simulink model "parte5_eje1_Ks"  (R2019b)
settings: Solver=VariableStepAuto  StartTime=0.0  StopTime=200  RelTol=1e-3
values from neighbouring files (symbols this model uses):
  H = 6.175    [parte5_ej2_GEPs_data0228.m]    (also in parte5_eje2_sintonizacionPSS.m = Syn.con(N_Gen,18)/2)
  Kd = 0    [parte5_ej2_GEPs_data0228.m]    (also in parte5_eje2_sintonizacionPSS.m = Syn.con(N_Gen,19))
  Ks = (Eb*Eqo)/(xd+xe)*cos(tho)    [parte5_eje2_sintonizacionPSS.m]
  RT = ra    [parte5_eje2_sintonizacionPSS.m]
  Te = 0.01    [parte5_ej2_GEPs_data0228.m]
  Tw = 3.5    [parte5_ej1_PSS_0228.m]    (also in parte5_eje1_caracteristicasPSS.m = Twt(i))
undefined symbols (not defined in the file or in its folder): Rp, Tg, Tp, TR
settings Model: Creator=cjuar  LastModifiedBy=cjuar

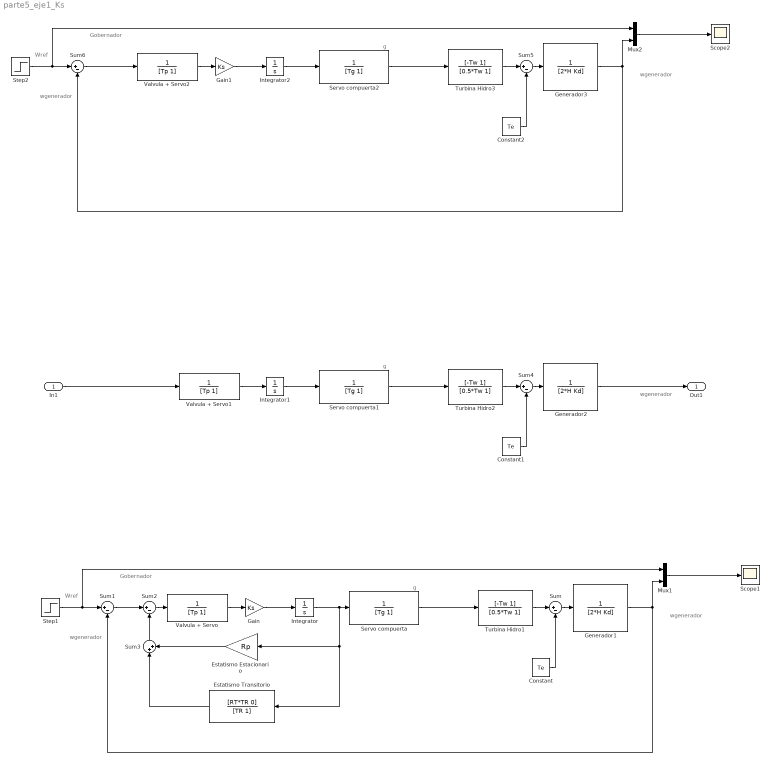
== system parte5_eje1_Ks ==
  note: Gobernador
  note: wgenerador
  note: g
  note: wgenerador
  note: Wref
  note: g
  note: wgenerador
  note: wgenerador
  note: Wref
  note: g
  note: Gobernador
  note: wgenerador
  In1 : Inport
  Constant : Constant  Value=Te
  Constant1 : Constant  Value=Te
  Constant2 : Constant  Value=Te
  Estatismo Estacionario : Gain  Gain=Rp
  Estatismo Transitorio : TransferFcn  Numerator=[RT*TR 0]  Denominator=[TR 1]
  Gain : Gain  Gain=Ks
  Gain1 : Gain  Gain=Ks
  Generador1 : TransferFcn  Denominator=[2*H Kd]
  Generador2 : TransferFcn  Denominator=[2*H Kd]
  Generador3 : TransferFcn  Denominator=[2*H Kd]
  Integrator : Integrator
  Integrator1 : Integrator
  Integrator2 : Integrator
  Mux1 : Mux  Inputs=2
  Mux2 : Mux  Inputs=2
  Scope1 : Scope
  Scope2 : Scope
  Servo compuerta : TransferFcn  Denominator=[Tg 1]
  Servo compuerta1 : TransferFcn  Denominator=[Tg 1]
  Servo compuerta2 : TransferFcn  Denominator=[Tg 1]
  Step1 : Step  After=0.1  SampleTime=0
  Step2 : Step  After=0.1  SampleTime=0
  Sum{,1..2,4..6} (6 alike) : Sum  Inputs=|+-
  Sum3 : Sum  Inputs=|++
  Turbina Hidro1 : TransferFcn  Numerator=[-Tw 1]  Denominator=[0.5*Tw 1]
  Turbina Hidro2 : TransferFcn  Numerator=[-Tw 1]  Denominator=[0.5*Tw 1]
  Turbina Hidro3 : TransferFcn  Numerator=[-Tw 1]  Denominator=[0.5*Tw 1]
  Valvula + Servo : TransferFcn  Denominator=[Tp 1]
  Valvula + Servo1 : TransferFcn  Denominator=[Tp 1]
  Valvula + Servo2 : TransferFcn  Denominator=[Tp 1]
  Out1 : Outport
  wires:
  Mux1/1 -> Scope1/1
  Sum1/1 -> Sum2/1
  Generador1/1 -> Mux1/2, Sum1/2
  Sum3/1 -> Sum2/2
  Estatismo Transitorio/1 -> Sum3/1
  Valvula + Servo/1 -> Gain/1
  Step1/1 -> Mux1/1, Sum1/1
  Estatismo Estacionario/1 -> Sum3/2
  Sum2/1 -> Valvula + Servo/1
  Gain/1 -> Integrator/1
  Turbina Hidro1/1 -> Sum/1
  Sum/1 -> Generador1/1
  Constant/1 -> Sum/2
  Integrator/1 -> Estatismo Estacionario/1, Estatismo Transitorio/1, Servo compuerta/1
  Servo compuerta/1 -> Turbina Hidro1/1
  In1/1 -> Valvula + Servo1/1
  Servo compuerta1/1 -> Turbina Hidro2/1
  Sum4/1 -> Generador2/1
  Constant1/1 -> Sum4/2
  Integrator1/1 -> Servo compuerta1/1
  Turbina Hidro2/1 -> Sum4/1
  Valvula + Servo1/1 -> Integrator1/1
  Generador2/1 -> Out1/1
  Sum6/1 -> Valvula + Servo2/1
  Step2/1 -> Mux2/1, Sum6/1
  Generador3/1 -> Mux2/2, Sum6/2
  Valvula + Servo2/1 -> Gain1/1
  Mux2/1 -> Scope2/1
  Servo compuerta2/1 -> Turbina Hidro3/1
  Sum5/1 -> Generador3/1
  Gain1/1 -> Integrator2/1
  Constant2/1 -> Sum5/2
  Integrator2/1 -> Servo compuerta2/1
  Turbina Hidro3/1 -> Sum5/1
